simulink model "manipulador_tray"  (R2015a)
settings: Solver=ode45  StartTime=0.0  StopTime=200  RelTol=1e-3
undefined symbols (not defined in the file or in its folder): tipo_control, tipo_tray
libraries: simulink x6
settings Model: Creator=Juan Esteban  LastModifiedBy=Juan Esteban

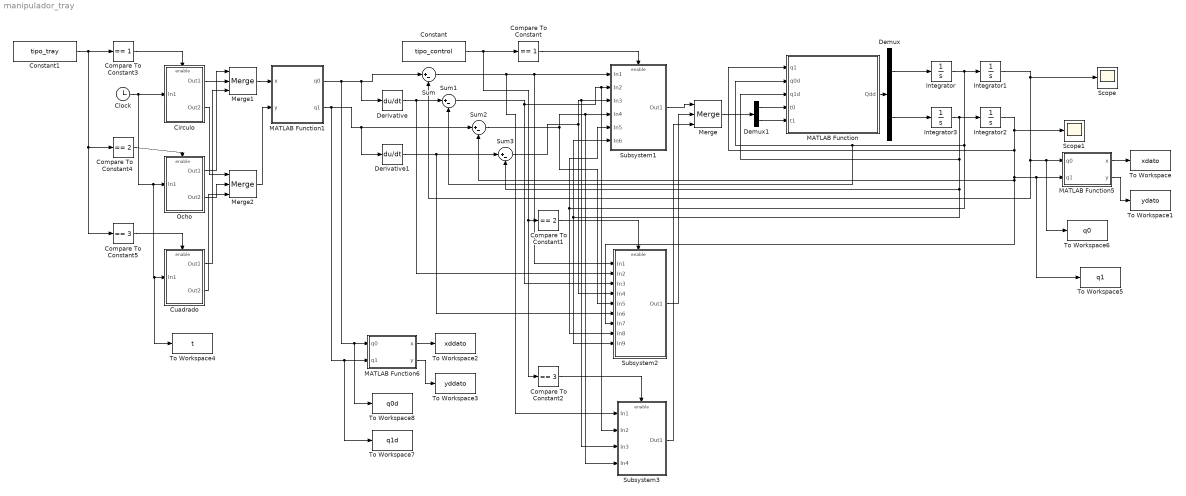
== system manipulador_tray ==
  Circulo : Subsystem
  Clock : Clock
  Compare To Constant : simulink/Logic and Bit Operations/Compare To Constant  relop===  const=1  OutDataTypeStr=boolean
  Compare To Constant1 : simulink/Logic and Bit Operations/Compare To Constant  relop===  const=2  OutDataTypeStr=boolean
  Compare To Constant2 : simulink/Logic and Bit Operations/Compare To Constant  relop===  const=3  OutDataTypeStr=boolean
  Compare To Constant3 : simulink/Logic and Bit Operations/Compare To Constant  relop===  const=1  OutDataTypeStr=boolean
  Compare To Constant4 : simulink/Logic and Bit Operations/Compare To Constant  relop===  const=2  OutDataTypeStr=boolean
  Compare To Constant5 : simulink/Logic and Bit Operations/Compare To Constant  relop===  const=3  OutDataTypeStr=boolean
  Constant : Constant  Value=tipo_control
  Constant1 : Constant  Value=tipo_tray
  Cuadrado : Subsystem
  Demux : Demux  Outputs=2
  Demux1 : Demux  Outputs=2
  Derivative : Derivative
  Derivative1 : Derivative
  Integrator{,1..3} (4 alike) : Integrator
  MATLAB Function : MATLAB Function  TreatAsAtomicUnit=on
  MATLAB Function1 : MATLAB Function  TreatAsAtomicUnit=on
  MATLAB Function5 : MATLAB Function  TreatAsAtomicUnit=on
  MATLAB Function6 : MATLAB Function  TreatAsAtomicUnit=on
  Merge : Merge  Inputs=3
  Merge1 : Merge  Inputs=3
  Merge2 : Merge  Inputs=3
  Ocho : Subsystem
  Scope : Scope
  Scope1 : Scope
  Subsystem1 : Subsystem
  Subsystem2 : Subsystem
  Subsystem3 : Subsystem
  Sum{,1..3} (4 alike) : Sum  Inputs=|+-
  To Workspace : ToWorkspace  VariableName=xdato  SampleTime=-1
  To Workspace1 : ToWorkspace  VariableName=ydato  SampleTime=-1
  To Workspace2 : ToWorkspace  VariableName=xddato  SampleTime=-1
  To Workspace3 : ToWorkspace  VariableName=yddato  SampleTime=-1
  To Workspace4 : ToWorkspace  VariableName=t  SampleTime=-1
  To Workspace5 : ToWorkspace  VariableName=q1  SampleTime=-1
  To Workspace6 : ToWorkspace  VariableName=q0  SampleTime=-1
  To Workspace7 : ToWorkspace  VariableName=q1d  SampleTime=-1
  To Workspace8 : ToWorkspace  VariableName=q0d  SampleTime=-1
  wires:
  MATLAB Function/1(Qdd) -> Demux/1
  Demux/1 -> Integrator/1
  Demux/2 -> Integrator3/1
  Integrator/1 -> Subsystem2/8(In8), Subsystem1/5(In5), Sum1/2, MATLAB Function/2(q0d), Integrator1/1
  Integrator3/1 -> Subsystem2/9(In9), Subsystem1/6(In6), Sum3/2, MATLAB Function/3(q1d), Integrator2/1
  Integrator2/1 -> Scope1/1, Subsystem2/7(In7), Sum2/2, To Workspace5/1, MATLAB Function5/2(q1), MATLAB Function/1(q1)
  Integrator1/1 -> Scope/1, To Workspace6/1, MATLAB Function5/1(q0), Sum/2
  Demux1/1 -> MATLAB Function/4(t0)
  Demux1/2 -> MATLAB Function/5(t1)
  Sum3/1 -> Subsystem2/4(In4), Subsystem3/3(In3), Subsystem1/3(In3)
  Sum2/1 -> Subsystem2/5(In5), Subsystem3/4(In4), Subsystem1/4(In4)
  Sum1/1 -> Subsystem2/3(In3), Subsystem3/2(In2), Subsystem1/2(In2)
  Sum/1 -> Subsystem3/1(In1), Subsystem2/1(In1), Subsystem1/1(In1)
  Derivative/1 -> Subsystem2/2(In2), Sum1/1
  Derivative1/1 -> Subsystem2/6(In6), Sum3/1
  MATLAB Function5/1(x) -> To Workspace/1
  MATLAB Function5/2(y) -> To Workspace1/1
  MATLAB Function6/2(y) -> To Workspace3/1
  MATLAB Function6/1(x) -> To Workspace2/1
  Merge/1 -> Demux1/1
  Subsystem1/1(Out1) -> Merge/1
  Subsystem2/1(Out1) -> Merge/2
  Constant/1 -> Compare To Constant1/1, Compare To Constant2/1, Compare To Constant/1
  Compare To Constant/1 -> Subsystem1/Enable
  Compare To Constant1/1 -> Subsystem2/Enable
  Subsystem3/1(Out1) -> Merge/3
  Compare To Constant2/1 -> Subsystem3/Enable
  Clock/1 -> To Workspace4/1, Cuadrado/1(In1), Ocho/1(In1), Circulo/1(In1)
  MATLAB Function1/1(q0) -> To Workspace8/1, MATLAB Function6/1(q0), Derivative/1, Sum/1
  MATLAB Function1/2(q1) -> To Workspace7/1, MATLAB Function6/2(q1), Derivative1/1, Sum2/1
  Constant1/1 -> Compare To Constant5/1, Compare To Constant4/1, Compare To Constant3/1
  Compare To Constant3/1 -> Circulo/Enable
  Merge1/1 -> MATLAB Function1/1(x)
  Circulo/1(Out1) -> Merge1/1
  Ocho/1(Out1) -> Merge1/2
  Circulo/2(Out2) -> Merge2/1
  Ocho/2(Out2) -> Merge2/2
  Merge2/1 -> MATLAB Function1/2(y)
  Compare To Constant4/1 -> Ocho/Enable
  Cuadrado/1(Out1) -> Merge1/3
  Cuadrado/2(Out2) -> Merge2/3
  Compare To Constant5/1 -> Cuadrado/Enable

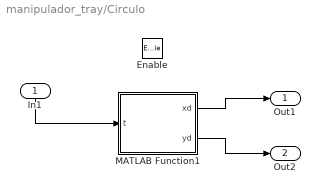
== system manipulador_tray/Circulo ==
  In1 : Inport
  Enable : EnablePort
  MATLAB Function1 : MATLAB Function  TreatAsAtomicUnit=on
  Out1 : Outport
  Out2 : Outport  Port=2
  wires:
  MATLAB Function1/1(xd) -> Out1/1
  MATLAB Function1/2(yd) -> Out2/1
  In1/1 -> MATLAB Function1/1(t)

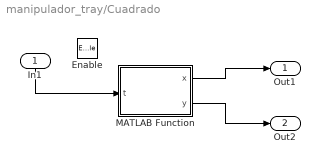
== system manipulador_tray/Cuadrado ==
  In1 : Inport
  Enable : EnablePort
  MATLAB Function : MATLAB Function  TreatAsAtomicUnit=on
  Out1 : Outport
  Out2 : Outport  Port=2
  wires:
  MATLAB Function/1(x) -> Out1/1
  MATLAB Function/2(y) -> Out2/1
  In1/1 -> MATLAB Function/1(t)

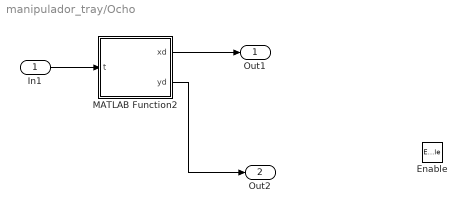
== system manipulador_tray/Ocho ==
  In1 : Inport
  Enable : EnablePort
  MATLAB Function2 : MATLAB Function  TreatAsAtomicUnit=on
  Out1 : Outport
  Out2 : Outport  Port=2
  wires:
  MATLAB Function2/2(yd) -> Out2/1
  MATLAB Function2/1(xd) -> Out1/1
  In1/1 -> MATLAB Function2/1(t)

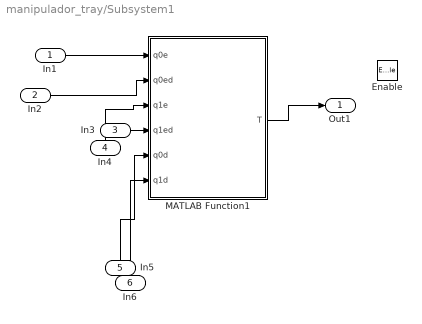
== system manipulador_tray/Subsystem1 ==
  In1 : Inport
  In2 : Inport  Port=2
  In3 : Inport  Port=3
  In4 : Inport  Port=4
  In5 : Inport  Port=5
  In6 : Inport  Port=6
  Enable : EnablePort
  MATLAB Function1 : MATLAB Function  TreatAsAtomicUnit=on
  Out1 : Outport
  wires:
  In5/1 -> MATLAB Function1/5(q0d)
  In4/1 -> MATLAB Function1/3(q1e)
  In6/1 -> MATLAB Function1/6(q1d)
  In1/1 -> MATLAB Function1/1(q0e)
  In2/1 -> MATLAB Function1/2(q0ed)
  In3/1 -> MATLAB Function1/4(q1ed)
  MATLAB Function1/1(T) -> Out1/1

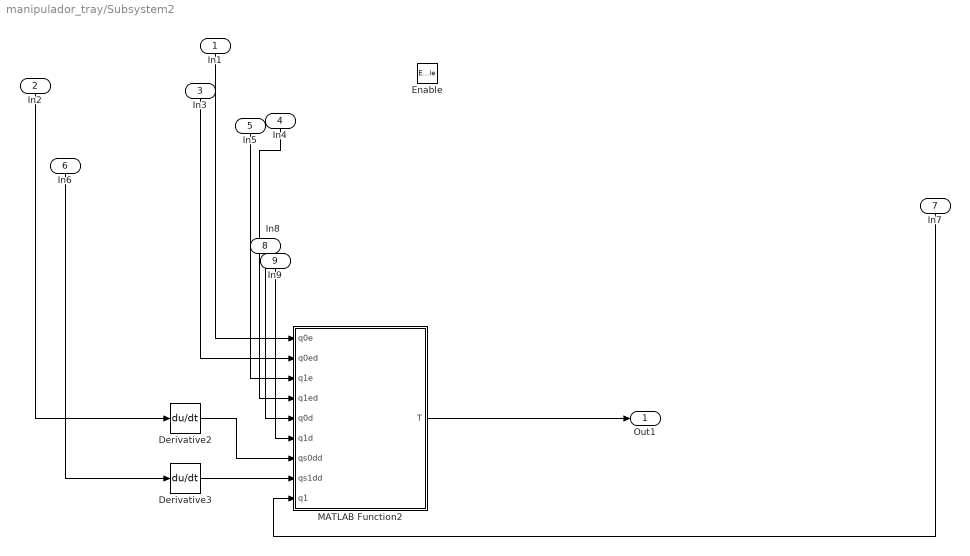
== system manipulador_tray/Subsystem2 ==
  In1 : Inport
  In2 : Inport  Port=2
  In3 : Inport  Port=3
  In4 : Inport  Port=4
  In5 : Inport  Port=5
  In6 : Inport  Port=6
  In7 : Inport  Port=7
  In8 : Inport  Port=8
  In9 : Inport  Port=9
  Enable : EnablePort
  Derivative2 : Derivative
  Derivative3 : Derivative
  MATLAB Function2 : MATLAB Function  TreatAsAtomicUnit=on
  Out1 : Outport
  wires:
  In9/1 -> MATLAB Function2/6(q1d)
  In3/1 -> MATLAB Function2/2(q0ed)
  In6/1 -> Derivative3/1
  In4/1 -> MATLAB Function2/4(q1ed)
  In5/1 -> MATLAB Function2/3(q1e)
  In7/1 -> MATLAB Function2/9(q1)
  In1/1 -> MATLAB Function2/1(q0e)
  In2/1 -> Derivative2/1
  In8/1 -> MATLAB Function2/5(q0d)
  MATLAB Function2/1(T) -> Out1/1
  Derivative3/1 -> MATLAB Function2/8(qs1dd)
  Derivative2/1 -> MATLAB Function2/7(qs0dd)

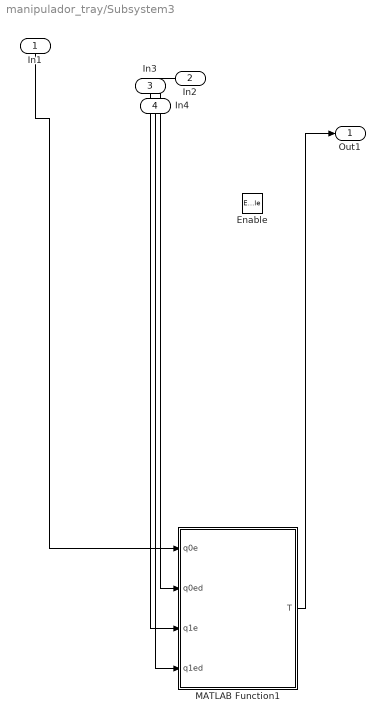
== system manipulador_tray/Subsystem3 ==
  In1 : Inport
  In2 : Inport  Port=2
  In3 : Inport  Port=3
  In4 : Inport  Port=4
  Enable : EnablePort
  MATLAB Function1 : MATLAB Function  TreatAsAtomicUnit=on
  Out1 : Outport
  wires:
  In4/1 -> MATLAB Function1/4(q1ed)
  In2/1 -> MATLAB Function1/2(q0ed)
  In1/1 -> MATLAB Function1/1(q0e)
  In3/1 -> MATLAB Function1/3(q1e)
  MATLAB Function1/1(T) -> Out1/1

== matlab function manipulador_tray/Subsystem1/MATLAB Function1 ==
  data: q0e input; T output; q0ed input; q1e input; q1ed input; q0d input; q1d input
function T = fcn(q0e,q0ed,q1e,q1ed,q0d,q1d)
F=[1.0256*sign(q0d);1.7842*sign(q1d)];
kp=[400 0;0 380];
kd=[1 0;0 1];
qe=[q0e;q1e];
qed=[q0ed;q1ed];
T=kp*qe+kd*qed+F;

== matlab function manipulador_tray/MATLAB Function ==
  data: q1 input; Qdd output; q0d input; q1d input; t0 input; t1 input
function Qdd = fcn(q1,q0d,q1d,t0,t1)
%#codegen
M=[1.7277+0.1908*cos(q1) 0.0918+0.0954*cos(q1);
    0.0918+0.0954*cos(q1) 0.9184];
C=[31.8142-0.0954*sin(q1)*q1d -0.0954*sin(q1)*(q0d+q1d);
    0.3418*sin(q1)*q0d 12.5783];
F=[1.0256*sign(q0d);1.7842*sign(q1d)];
T=[t0;t1];
Qd=[q0d;q1d];
Qdd=inv(M)*(T-C*Qd-F);

== matlab function manipulador_tray/MATLAB Function1 ==
  data: x input; q0 output; y input; q1 output
function [q0,q1] = fcn(x,y)

l1 = 0.445;
l2 = 0.355;

% l1 = 10;
% l2 = 10;

% l1 = 8;
% l2 = 8;
 
% q = (-2*y*R + (sqrt(x^2 + y^2 - (r-R)^2))*(sqrt(-x^2 - y^2 + (r+R)^2)))/((y-r)*(y+r)+(x-R)^2);
% 
% s = -(sqrt(-x^2 - y^2 + (r+R)^2))/(sqrt(x^2 + y^2 - (r-R)^2));
% 
% q0 = 2*atan(q) + pi;
% q1 = 2*atan(s) + pi;

% if x<0 
    q0 = pi/2 - acos((l1^2-l2^2+x^2+y^2)/(2*l1*sqrt(x^2+y^2))) - atan2(y,x);%asin(x/sqrt(x^2+y^2));
    q1 = acos((x^2+y^2-l1^2-l2^2)/(2*l1*l2));
% else 
%     q0 = pi/2 - acos((l1^2-(l2^2)+x^2+y^2)/(2*l1*sqrt(x^2+y^2))) - acos(x/sqrt(x^2+y^2));
%     q1 = acos((x^2+y^2-(l1^2)-(l2^2))/(2*l1*l2));
% end

== matlab function manipulador_tray/Cuadrado/MATLAB Function ==
  data: x output; t input; y output
function [x,y] = fcn(t)

if t <= 25 
    y = 0.55;
    x = -0.002*t+0.05;
elseif t <= 75
    y = -0.002*t+0.6;
    x = -0.05;
elseif t <= 125
    y = 0.45;
    x = 0.002*t-0.2;
elseif t <= 175
    y = 0.002*t+0.2;
    x = 0.05;
elseif t <= 200
    y = 0.55;
    x = -0.002*t+0.4;
else
    y=0.55;
    x=0;
end

== matlab function manipulador_tray/MATLAB Function5 ==
  data: x output; q0 input; y output; q1 input
function [x,y] = fcn(q0,q1)
%#codegen
x=0.445*cos(q0)+0.355*cos(q1+q0);
y=0.445*sin(q0)+0.355*sin(q1+q0);

== matlab function manipulador_tray/MATLAB Function6 ==
  data: x output; q0 input; y output; q1 input
function [x,y] = fcn(q0,q1)
%#codegen
x=0.445*cos(q0)+0.355*cos(q1+q0);
y=0.445*sin(q0)+0.355*sin(q1+q0);

== matlab function manipulador_tray/Subsystem2/MATLAB Function2 ==
  data: q0e input; T output; q0ed input; q1e input; q1ed input; q0d input; q1d input; qs0dd input; qs1dd input; q1 input
function T = fcn(q0e,q0ed,q1e,q1ed,q0d,q1d,qs0dd,qs1dd,q1)
M=[1.7277+0.1908*cos(q1) 0.0918+0.0954*cos(q1);
    0.0918+0.0954*cos(q1) 0.9184];
C=[31.8142-0.0954*sin(q1)*q1d -0.0954*sin(q1)*(q0d+q1d);
    0.3418*sin(q1)*q0d 12.5783];
F=[1.0256*sign(q0d);1.7842*sign(q1d)];
kp=[1 0; 0 1];
kd=[10000 0; 0 10000];
qe=[q0e;q1e];
qed=[q0ed;q1ed];
qd=[q0d;q1d];
qsdd=[qs0dd;qs1dd];
a=qsdd+kd*qed+kp*qe;
T=0.003*M*a+C*qd+F;

== matlab function manipulador_tray/Subsystem3/MATLAB Function1 ==
  data: q0e input; T output; q0ed input; q1e input; q1ed input
function T = fcn(q0e,q0ed,q1e,q1ed)
kp=[4000 0;0 3800];
kd=[10000 0;0 10000];
qe=[q0e;q1e];
qed=[q0ed;q1ed];
T=kp*qe+kd*qed;

== matlab function manipulador_tray/Ocho/MATLAB Function2 ==
  data: t input; xd output; yd output
function [xd,yd] = ruta3(t)
%#codegen
        cv = 20;
        xd = 0.1*sin(t/(0.5*cv)); %2*t(k);  
        yd = 0.1*cos(t/(cv))+0.7;

== matlab function manipulador_tray/Circulo/MATLAB Function1 ==
  data: t input; xd output; yd output
function [xd,yd] = ruta1(t)
%#codegen
        cv = 20;
        xd = 0.1*sin(t/(cv)); %2*t(k);  
        yd = 0.1*cos(t/(cv))+0.7;
